simulink model "fuzzy_pid"  (R2022a)
settings: Solver=VariableStepAuto  StartTime=0.0  StopTime=5  RelTol=1e-3
values from neighbouring files (symbols this model uses):
  d = -0.008    [parameter.m]
  i = i-1    [FuzzyPID.m]    (also in parameter.m = 0.03)
  Ke = 3    [parameter.m]
  Kec = 1.5    [parameter.m]
  Kp = 0.0075    [parameter.m]
  Ks = 100    [parameter.m]
  p = 0.7    [parameter.m]
libraries: slpidlib x2, fuzblock x1
settings Model: Creator=li_fe  LastModifiedBy=li_fe

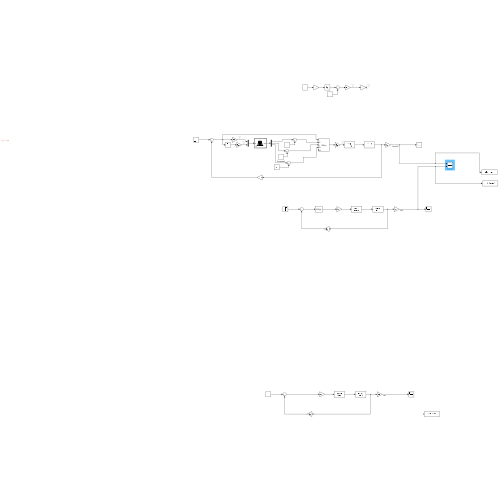
[thumbnail: Simulink's stored preview of the top-level diagram]
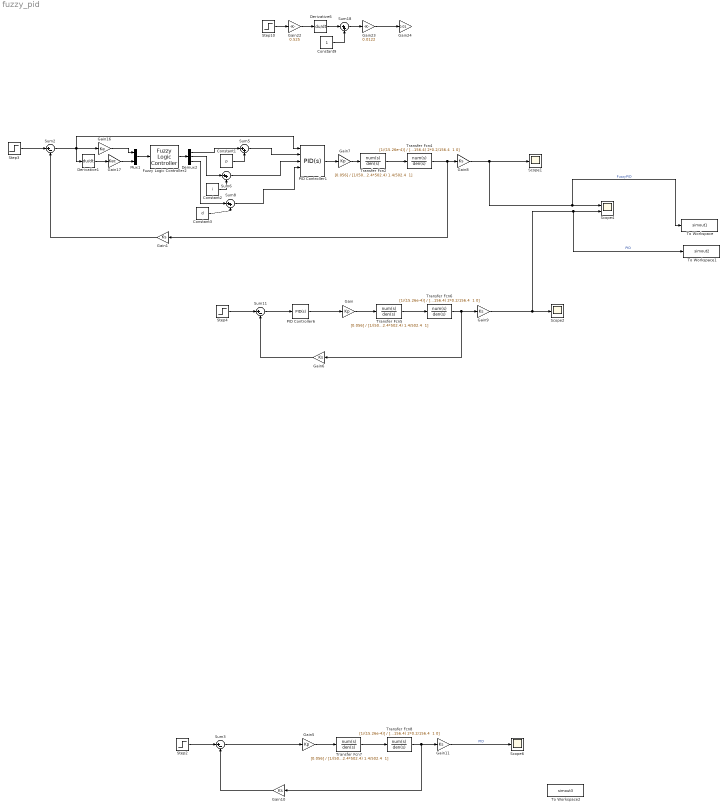
== system fuzzy_pid ==
  Constant1 : Constant  Value=p
  Constant2 : Constant  Value=i
  Constant3 : Constant  Value=d
  Constant9 : Constant
  Demux2 : Demux  Outputs=3
  Derivative1 : Derivative
  Derivative6 : Derivative
  Fuzzy Logic Controller2 : fuzblock/Fuzzy Logic  Controller  FIS='Fuzzy_Pid.fis'  OutputSampleNumber=101  DataType=double  FuzzifiedInputs=off  RuleFiringStrengths=off  RuleOutputs=off  AggregatedOutputs=off  SimulateUsing=Interpreted execution  OutOfRangeInputValueMessage=warning  NoRuleFiredMessage=warning  EmptyOutputFuzzySetMessage=warning
  Gain : Gain  Gain=Kp
  Gain{1,6,8..11} (6 alike) : Gain  Gain=Ks
  Gain16 : Gain  Gain=Ke
  Gain17 : Gain  Gain=Kec
  Gain22 : Gain  Gain=0.525
  Gain23 : Gain  Gain=0.0122
  Gain24 : Gain  Gain=0.01
  Gain5 : Gain  Gain=Kp
  Gain7 : Gain  Gain=Kp
  Mux1 : Mux  Inputs=2
  PID Controller1 : slpidlib/PID Controller  Controller=PID  Form=Parallel  TimeDomain=Continuous-time  UseExternalTs=off  SampleTime=-1  IntegratorMethod=Forward Euler  FilterMethod=Forward Euler  ControllerParametersSource=external  P=1  I=1  UseKiTs=off  D=1  N=100  UseFilter=on  TunerSelectOption=Transfer Function Based (PID Tuner App)  InitialConditionSource=internal  InitialConditionForIntegrator=0  InitialConditionForFilter=0  DifferentiatorICPrevScaledInput=0  ExternalReset=none  TrackingMode=off  Kt=1  LimitOutput=off  SatLimitsSource=internal  UpperSaturationLimit=inf  LowerSaturationLimit=-inf  LinearizeAsGain=on  AntiWindupMode=none  Kb=1  POutMin=[]  POutMax=[]  IOutMin=[]  IOutMax=[]  DOutMin=[]  DOutMax=[]  NOutMin=[]  NOutMax=[]  SumOutMin=[]  SumOutMax=[]  SaturationOutMin=[]  SaturationOutMax=[]  PParamMin=[]  PParamMax=[]  IParamMin=[]  IParamMax=[]  DParamMin=[]  DParamMax=[]  NParamMin=[]  NParamMax=[]  KbParamMin=[]  KbParamMax=[]  KtParamMin=[]  KtParamMax=[]  KbOutMin=[]  KbOutMax=[]  KtOutMin=[]  KtOutMax=[]  IntegratorOutMin=[]  IntegratorOutMax=[]  FilterOutMin=[]  FilterOutMax=[]  SumI1OutMin=[]  SumI1OutMax=[]  SumI2OutMin=[]  SumI2OutMax=[]  SumI3OutMin=[]  SumI3OutMax=[]  SumI4OutMin=[]  SumI4OutMax=[]  SumDOutMin=[]  SumDOutMax=[]  DifferentiatorOutMin=[]  DifferentiatorOutMax=[]  FilterDiffOutCoefMin=[]  FilterDiffOutCoefMax=[]  ReciprocalOutMin=[]  ReciprocalOutMax=[]  SumDenOutMin=[]  SumDenOutMax=[]  SumNumOutMin=[]  SumNumOutMax=[]  DivideOutMin=[]  DivideOutMax=[]  UdiffTsProdOutMin=[]  UdiffTsProdOutMax=[]  NTsProdOutMin=[]  NTsProdOutMax=[]  UintegralTsProdOutMin=[]  UintegralTsProdOutMax=[]  UngainTsProdOutMin=[]  UngainTsProdOutMax=[]  IntegratorContinuousStateAttributes=''  IntegratorStateMustResolveToSignalObject=off  IntegratorRTWStateStorageClass=Auto  FilterContinuousStateAttributes=''  FilterStateMustResolveToSignalObject=off  FilterRTWStateStorageClass=Auto  ParallelPVariant=ExternalParameters  IdealPVariant=Disabled  IVariant=ExternalParameters  DVariant=ExternalParameters  IntegratorVariant=Continuous  SatVariant=Disabled  AWVariant=Passthrough  PCopyVariant=Disabled  TRVariant=Disabled  FdbkBlocksVariant=Forward  IdealPFdbkVariant=Disabled  SatFdbkVariant=Disabled  DerivativeFilterVariant=ContFilter  NVariant=ExternalParameters  NCopyVariant=Disabled  FilterICVariant=InternalICsFilter  IntegratorICVariant=InternalICs  ExternalResetVariant=Disabled  TRSumVariant=Passthrough  SumFdbkVariant=Disabled  SumVariant=Sum_PID  TsampFilterVariant=InternalTs  TsampNgainVariant=Passthrough  TsampIntegralVariant=Passthrough  ExternalSaturationOutDataTypeStr=Inherit: Same as second input  aMode=0
  PID Controller6 : slpidlib/PID Controller  Controller=PID  Form=Parallel  TimeDomain=Continuous-time  UseExternalTs=off  SampleTime=-1  IntegratorMethod=Forward Euler  FilterMethod=Forward Euler  ControllerParametersSource=internal  P=0.7  I=0.03  UseKiTs=off  D=-0.088  N=3.44088549948957  UseFilter=on  TunerSelectOption=Transfer Function Based (PID Tuner App)  InitialConditionSource=internal  InitialConditionForIntegrator=0  InitialConditionForFilter=0  DifferentiatorICPrevScaledInput=0  ExternalReset=none  TrackingMode=off  Kt=1  LimitOutput=off  SatLimitsSource=internal  UpperSaturationLimit=inf  LowerSaturationLimit=-inf  LinearizeAsGain=on  AntiWindupMode=none  Kb=1  POutMin=[]  POutMax=[]  IOutMin=[]  IOutMax=[]  DOutMin=[]  DOutMax=[]  NOutMin=[]  NOutMax=[]  SumOutMin=[]  SumOutMax=[]  SaturationOutMin=[]  SaturationOutMax=[]  PParamMin=[]  PParamMax=[]  IParamMin=[]  IParamMax=[]  DParamMin=[]  DParamMax=[]  NParamMin=[]  NParamMax=[]  KbParamMin=[]  KbParamMax=[]  KtParamMin=[]  KtParamMax=[]  KbOutMin=[]  KbOutMax=[]  KtOutMin=[]  KtOutMax=[]  IntegratorOutMin=[]  IntegratorOutMax=[]  FilterOutMin=[]  FilterOutMax=[]  SumI1OutMin=[]  SumI1OutMax=[]  SumI2OutMin=[]  SumI2OutMax=[]  SumI3OutMin=[]  SumI3OutMax=[]  SumI4OutMin=[]  SumI4OutMax=[]  SumDOutMin=[]  SumDOutMax=[]  DifferentiatorOutMin=[]  DifferentiatorOutMax=[]  FilterDiffOutCoefMin=[]  FilterDiffOutCoefMax=[]  ReciprocalOutMin=[]  ReciprocalOutMax=[]  SumDenOutMin=[]  SumDenOutMax=[]  SumNumOutMin=[]  SumNumOutMax=[]  DivideOutMin=[]  DivideOutMax=[]  UdiffTsProdOutMin=[]  UdiffTsProdOutMax=[]  NTsProdOutMin=[]  NTsProdOutMax=[]  UintegralTsProdOutMin=[]  UintegralTsProdOutMax=[]  UngainTsProdOutMin=[]  UngainTsProdOutMax=[]  IntegratorContinuousStateAttributes=''  IntegratorStateMustResolveToSignalObject=off  IntegratorRTWStateStorageClass=Auto  FilterContinuousStateAttributes=''  FilterStateMustResolveToSignalObject=off  FilterRTWStateStorageClass=Auto  ParallelPVariant=InternalParameters  IdealPVariant=Disabled  IVariant=InternalParameters  DVariant=InternalParameters  IntegratorVariant=Continuous  SatVariant=Disabled  AWVariant=Passthrough  PCopyVariant=Disabled  TRVariant=Disabled  FdbkBlocksVariant=Forward  IdealPFdbkVariant=Disabled  SatFdbkVariant=Disabled  DerivativeFilterVariant=ContFilter  NVariant=InternalParameters  NCopyVariant=Disabled  FilterICVariant=InternalICsFilter  IntegratorICVariant=InternalICs  ExternalResetVariant=Disabled  TRSumVariant=Passthrough  SumFdbkVariant=Disabled  SumVariant=Sum_PID  TsampFilterVariant=InternalTs  TsampNgainVariant=Passthrough  TsampIntegralVariant=Passthrough  ExternalSaturationOutDataTypeStr=Inherit: Same as second input  aMode=0
  Scope1 : Scope
  Scope2 : Scope
  Scope4 : Scope  NumInputPorts=2
  Scope6 : Scope
  Step{2..4,10} (4 alike) : Step  SampleTime=0
  Sum11 : Sum  Inputs=|+-
  Sum{5..6,8,18} (4 alike) : Sum  Inputs=|++
  Sum2 : Sum  Inputs=|+-
  Sum3 : Sum  Inputs=|+-
  To Workspace : ToWorkspace  VariableName=simout1  SaveFormat=Timeseries  SampleTime=-1
  To Workspace1 : ToWorkspace  VariableName=simout2  SaveFormat=Timeseries  SampleTime=-1
  To Workspace2 : ToWorkspace  VariableName=simout3  SaveFormat=Timeseries  SampleTime=-1
  Transfer Fcn2 : TransferFcn  Numerator=[0.056]  Denominator="[1/(502.4*502.4) 1.4/502.4  1]"
  Transfer Fcn4 : TransferFcn  Numerator=[1/(15.26e-4)]  Denominator="[1/(156.4*156.4) 2*0.2/156.4  1 0]"
  Transfer Fcn5 : TransferFcn  Numerator=[0.056]  Denominator="[1/(502.4*502.4) 1.4/502.4  1]"
  Transfer Fcn6 : TransferFcn  Numerator=[1/(15.26e-4)]  Denominator="[1/(156.4*156.4) 2*0.2/156.4  1 0]"
  Transfer Fcn7 : TransferFcn  Numerator=[0.056]  Denominator="[1/(502.4*502.4) 1.4/502.4  1]"
  Transfer Fcn8 : TransferFcn  Numerator=[1/(15.26e-4)]  Denominator="[1/(156.4*156.4) 2*0.2/156.4  1 0]"
  wires:
  ? -> ?
  Fuzzy Logic Controller2/1 -> Demux2/1
  Mux1/1 -> Fuzzy Logic Controller2/1
  Derivative1/1 -> Gain17/1
  Sum2/1 -> PID Controller1/1, Derivative1/1, Gain16/1
  Step3/1 -> Sum2/1
  Sum8/1 -> PID Controller1/4
  Sum6/1 -> PID Controller1/3
  Demux2/1 -> Sum5/1
  Sum5/1 -> PID Controller1/2
  Demux2/2 -> Sum6/1
  Demux2/3 -> Sum8/1
  Constant1/1 -> Sum5/2
  Constant2/1 -> Sum6/2
  Constant3/1 -> Sum8/2
  Gain1/1 -> Sum2/2
  Gain6/1 -> Sum11/2
  Gain7/1 -> Transfer Fcn2/1
  PID Controller1/1 -> Gain7/1
  Transfer Fcn4/1 -> Gain8/1, Gain1/1
  PID Controller6/1 -> Gain/1
  Gain/1 -> Transfer Fcn5/1
  Gain8/1 -> To Workspace/1, Scope4/1, Scope1/1  "FuzzyPID"
  Step4/1 -> Sum11/1
  Transfer Fcn6/1 -> Gain9/1, Gain6/1
  Sum11/1 -> PID Controller6/1
  Gain16/1 -> Mux1/1
  Gain17/1 -> Mux1/2
  Transfer Fcn5/1 -> Transfer Fcn6/1
  Transfer Fcn2/1 -> Transfer Fcn4/1
  Derivative6/1 -> Sum18/1
  Constant9/1 -> Sum18/2
  Step10/1 -> Gain22/1
  Gain22/1 -> Derivative6/1
  Sum18/1 -> Gain23/1
  Gain23/1 -> Gain24/1
  Gain9/1 -> To Workspace1/1, Scope4/2, Scope2/1  "PID"
  Gain11/1 -> Scope6/1  "PID"
  Gain10/1 -> Sum3/2
  Transfer Fcn8/1 -> Gain11/1, Gain10/1
  Step2/1 -> Sum3/1
  Gain5/1 -> Transfer Fcn7/1
  Transfer Fcn7/1 -> Transfer Fcn8/1
  Sum3/1 -> Gain5/1
